simulink model "lab3Simu"  (R2021b)
settings: Solver=VariableStepAuto  StartTime=0.0  StopTime=15  RelTol=1e-3
settings Model: Creator=14571525  LastModifiedBy=14571525

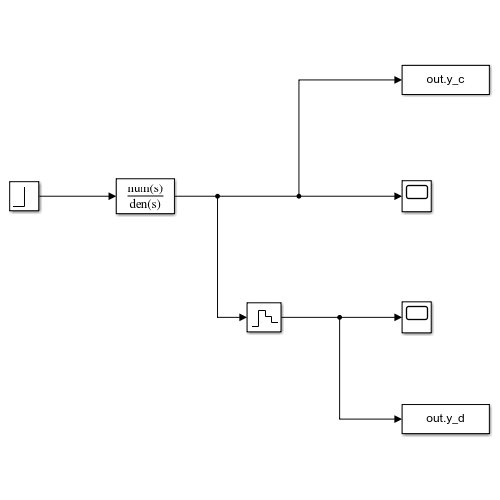
[thumbnail: Simulink's stored preview of the top-level diagram]
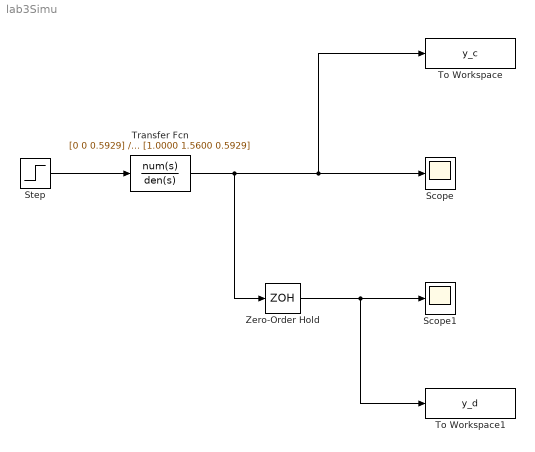
== system lab3Simu ==
  Scope : Scope
  Scope1 : Scope
  Step : Step  Time=0  After=1.17  SampleTime=0
  To Workspace : ToWorkspace  VariableName=y_c  SaveFormat=Timeseries  SampleTime=-1
  To Workspace1 : ToWorkspace  VariableName=y_d  SaveFormat=Timeseries  SampleTime=-1
  Transfer Fcn : TransferFcn  Numerator=[0 0 0.5929]  Denominator=[1.0000 1.5600 0.5929]
  Zero-Order Hold : ZeroOrderHold  SampleTime=1.2939
  wires:
  Step/1 -> Transfer Fcn/1
  Transfer Fcn/1 -> Zero-Order Hold/1, Scope/1, To Workspace/1
  Zero-Order Hold/1 -> To Workspace1/1, Scope1/1
